simulink model "simple_ST"  (R2022b)
settings: Solver=ode1  StartTime=0.0  StopTime=30  FixedStep=0.01  RelTol=1e-3
settings Model: Creator=Adan Daniel  LastModifiedBy=Adan Daniel

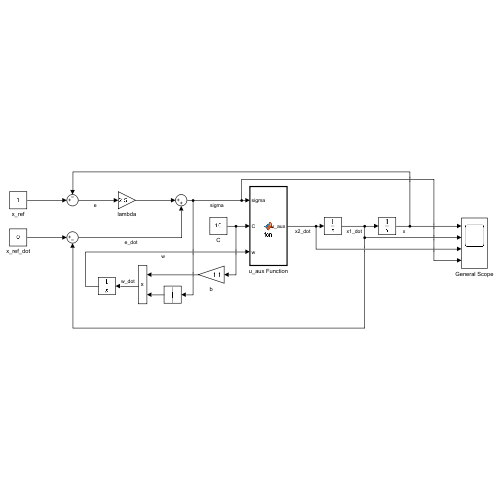
[thumbnail: Simulink's stored preview of the top-level diagram]
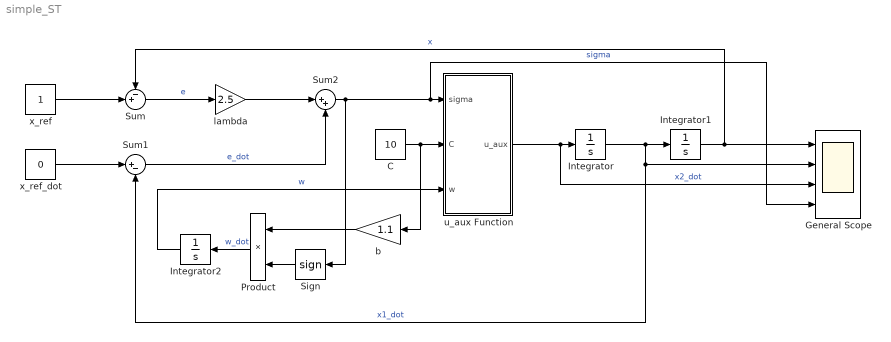
== system simple_ST ==
  C : Constant  Value=10
  General Scope : Scope  NumInputPorts=4
  Integrator : Integrator
  Integrator1 : Integrator
  Integrator2 : Integrator
  Product : Product
  Sign : Signum
  Sum : Sum  Inputs=-+|
  Sum1 : Sum  Inputs=|+-
  Sum2 : Sum  Inputs=|++
  b : Gain  Gain=1.1
  lambda : Gain  Gain=2.5
  u_aux Function : MATLAB Function  TreatAsAtomicUnit=on
  x_ref : Constant
  x_ref_dot : Constant  Value=0
  wires:
  x_ref/1 -> Sum/2
  x_ref_dot/1 -> Sum1/1
  Sum/1 -> lambda/1  "e"
  Sum1/1 -> Sum2/2  "e_dot"
  lambda/1 -> Sum2/1
  Sum2/1 -> General Scope/4, u_aux Function/1(sigma), Sign/1  "sigma"
  C/1 -> b/1, u_aux Function/2(C)
  u_aux Function/1(u_aux) -> General Scope/3, Integrator/1  "x2_dot"
  Integrator/1 -> Integrator1/1, General Scope/2, Sum1/2  "x1_dot"
  Integrator1/1 -> General Scope/1, Sum/1  "x"
  Sign/1 -> Product/2
  b/1 -> Product/1
  Product/1 -> Integrator2/1  "w_dot"
  Integrator2/1 -> u_aux Function/3(w)  "w"

== matlab function simple_ST/u_aux Function ==
  data: sigma input; u_aux output; C input; w input
function u_aux = fcn(sigma, C, w)

%% Super-twisting constants

c = 1.5 * sqrt(C);
% b = 1.1 * C;

u_aux = c * (abs(sigma))^(0.5) * sign(sigma) + w;
